simulink model "part19"  (R2017b)
settings: Solver=VariableStepAuto  StartTime=0.0  StopTime=40  RelTol=1e-3
settings Model: Creator=admin  LastModifiedBy=admin

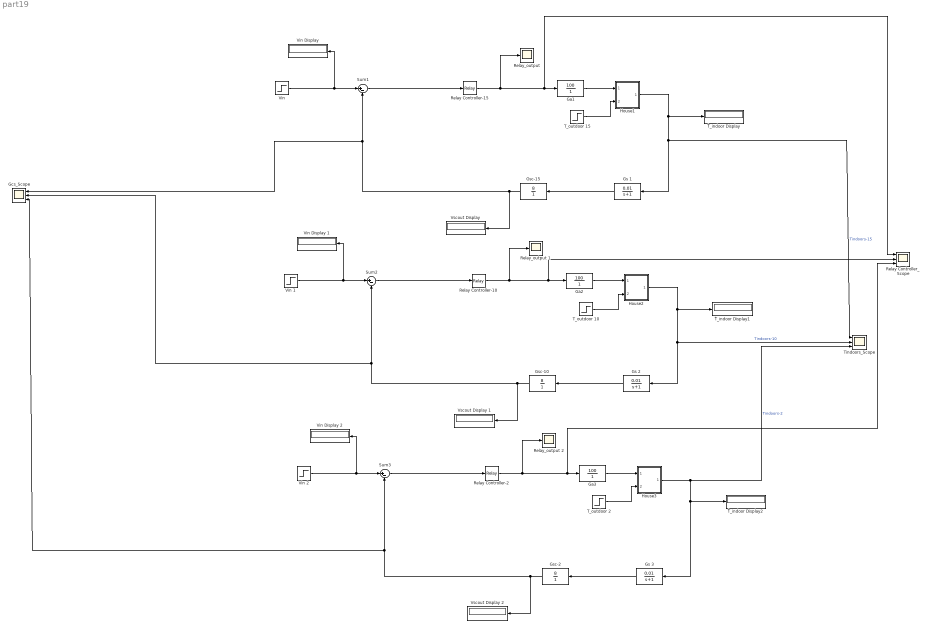
== system part19 ==
  Ga1 : TransferFcn  Numerator=[100]  Denominator=[1 ]
  Ga2 : TransferFcn  Numerator=[100]  Denominator=[1 ]
  Ga3 : TransferFcn  Numerator=[100]  Denominator=[1 ]
  "Gcs_Scope " : Scope  NumInputPorts=3
  Gs 1 : TransferFcn  Numerator=[0.01]  Denominator=[1 1]
  Gs 2 : TransferFcn  Numerator=[0.01]  Denominator=[1 1]
  Gs 3 : TransferFcn  Numerator=[0.01]  Denominator=[1 1]
  Gsc-10 : TransferFcn  Numerator=[8]  Denominator=[1 ]
  Gsc-15 : TransferFcn  Numerator=[8]  Denominator=[1 ]
  Gsc-2 : TransferFcn  Numerator=[8]  Denominator=[1 ]
  House1 : Subsystem
      mask Display: image(fullfile(matlabroot,'toolbox','simulink','simdemos','simgeneral','images','HouseHeatHousePix.svg'))
  House2 : Subsystem
      mask Display: image(fullfile(matlabroot,'toolbox','simulink','simdemos','simgeneral','images','HouseHeatHousePix.svg'))
  House3 : Subsystem
      mask Display: image(fullfile(matlabroot,'toolbox','simulink','simdemos','simgeneral','images','HouseHeatHousePix.svg'))
  Relay Controller-10 : Relay  OnSwitchValue=0.001  OffSwitchValue=-0.001  OnOutputValue=10
  Relay Controller-15 : Relay  OnSwitchValue=0.001  OffSwitchValue=-0.001  OnOutputValue=10
  Relay Controller-2 : Relay  OnSwitchValue=0.001  OffSwitchValue=-0.001  OnOutputValue=10
  "Relay Controller_Scope " : Scope  NumInputPorts=3
  "Relay_output " : Scope
  Relay_output 1 : Scope
  Relay_output 2 : Scope
  Sum1 : Sum  Inputs=|+-
  Sum2 : Sum  Inputs=|+-
  Sum3 : Sum  Inputs=|+-
  T_outdoor 10 : Step  Time=0  After=10  SampleTime=0
  "T_outdoor 15 " : Step  Time=0  After=15  SampleTime=0
  T_outdoor 2 : Step  Time=0  After=2  SampleTime=0
  "Tindoors_Scope " : Scope  NumInputPorts=3
  "Vin " : Step  Time=0  After=2.061  SampleTime=0
  Vin 1 : Step  Time=0  After=2.061  SampleTime=0
  Vin 2 : Step  Time=0  After=2.061  SampleTime=0
  "Vin Display " : Display
  Vin Display 1 : Display
  Vin Display 2 : Display
  "Vscout Display " : Display
  Vscout Display 1 : Display
  Vscout Display 2 : Display
  ْT_indoor Display : Display
  ْT_indoor Display1 : Display
  ْT_indoor Display2 : Display
  wires:
  "Vin "/1 -> "Vin Display "/1, Sum1/1
  Ga1/1 -> House1/1(Heater QDot In)
  Gs 1/1 -> Gsc-15/1
  Relay Controller-15/1 -> "Relay Controller_Scope "/1, Ga1/1, "Relay_output "/1
  Sum1/1 -> Relay Controller-15/1
  Gsc-15/1 -> "Gcs_Scope "/1, Sum1/2, "Vscout Display "/1
  "T_outdoor 15 "/1 -> House1/2(Outdoor Temp Tout)
  House1/1(Room Temp Troom) -> ْT_indoor Display/1, Gs 1/1, "Tindoors_Scope "/1  "Tindoors-15"
  Vin 1/1 -> Vin Display 1/1, Sum2/1
  Ga2/1 -> House2/1(Heater QDot In)
  Gs 2/1 -> Gsc-10/1
  Relay Controller-10/1 -> "Relay Controller_Scope "/2, Ga2/1, Relay_output 1/1
  Sum2/1 -> Relay Controller-10/1
  Gsc-10/1 -> "Gcs_Scope "/2, Sum2/2, Vscout Display 1/1
  T_outdoor 10/1 -> House2/2(Outdoor Temp Tout)
  House2/1(Room Temp Troom) -> ْT_indoor Display1/1, "Tindoors_Scope "/2, Gs 2/1  "Tindoors-10"
  Vin 2/1 -> Vin Display 2/1, Sum3/1
  Ga3/1 -> House3/1(Heater QDot In)
  Gs 3/1 -> Gsc-2/1
  Relay Controller-2/1 -> "Relay Controller_Scope "/3, Ga3/1, Relay_output 2/1
  Sum3/1 -> Relay Controller-2/1
  Gsc-2/1 -> "Gcs_Scope "/3, Sum3/2, Vscout Display 2/1
  T_outdoor 2/1 -> House3/2(Outdoor Temp Tout)
  House3/1(Room Temp Troom) -> "Tindoors_Scope "/3, ْT_indoor Display2/1, Gs 3/1  "Tindoors-2"

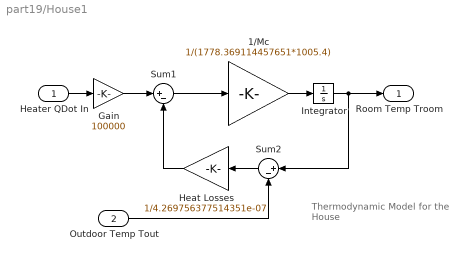
== system part19/House1 ==
  note: Thermodynamic Model
      | for the House
  Heater QDot In : Inport
  Outdoor Temp Tout : Inport  Port=2
  1/Mc : Gain  Gain=1/(1778.369114457651*1005.4)  SaturateOnIntegerOverflow=on  OutDataTypeStr=Inherit: Same as input  ParamDataTypeStr=Inherit: Same as input
  Gain : Gain  Gain=100000
  Heat Losses : Gain  Gain=1/4.269756377514351e-07  SaturateOnIntegerOverflow=on  OutDataTypeStr=Inherit: Same as input  ParamDataTypeStr=Inherit: Same as input
  Integrator : Integrator  InitialCondition=20
  Sum1 : Sum  Inputs=|+-  SaturateOnIntegerOverflow=on  InputSameDT=on  OutDataTypeStr=Inherit: Same as first input
  Sum2 : Sum  Inputs=|+-  SaturateOnIntegerOverflow=on  InputSameDT=on  OutDataTypeStr=Inherit: Same as first input
  Room Temp Troom : Outport  InitialOutput=0
  wires:
  Outdoor Temp Tout/1 -> Sum2/2
  Heater QDot In/1 -> Gain/1
  Sum1/1 -> 1/Mc/1
  Sum2/1 -> Heat Losses/1
  Heat Losses/1 -> Sum1/2
  1/Mc/1 -> Integrator/1
  Integrator/1 -> Sum2/1, Room Temp Troom/1
  Gain/1 -> Sum1/1

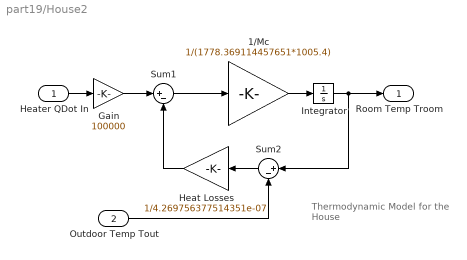
== system part19/House2 ==
  note: Thermodynamic Model
      | for the House
  Heater QDot In : Inport
  Outdoor Temp Tout : Inport  Port=2
  1/Mc : Gain  Gain=1/(1778.369114457651*1005.4)  SaturateOnIntegerOverflow=on  OutDataTypeStr=Inherit: Same as input  ParamDataTypeStr=Inherit: Same as input
  Gain : Gain  Gain=100000
  Heat Losses : Gain  Gain=1/4.269756377514351e-07  SaturateOnIntegerOverflow=on  OutDataTypeStr=Inherit: Same as input  ParamDataTypeStr=Inherit: Same as input
  Integrator : Integrator  InitialCondition=20
  Sum1 : Sum  Inputs=|+-  SaturateOnIntegerOverflow=on  InputSameDT=on  OutDataTypeStr=Inherit: Same as first input
  Sum2 : Sum  Inputs=|+-  SaturateOnIntegerOverflow=on  InputSameDT=on  OutDataTypeStr=Inherit: Same as first input
  Room Temp Troom : Outport  InitialOutput=0
  wires:
  Outdoor Temp Tout/1 -> Sum2/2
  Heater QDot In/1 -> Gain/1
  Sum1/1 -> 1/Mc/1
  Sum2/1 -> Heat Losses/1
  Heat Losses/1 -> Sum1/2
  1/Mc/1 -> Integrator/1
  Integrator/1 -> Sum2/1, Room Temp Troom/1
  Gain/1 -> Sum1/1

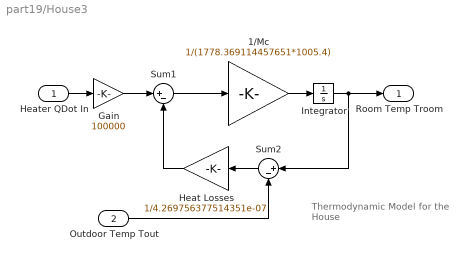
== system part19/House3 ==
  note: Thermodynamic Model
      | for the House
  Heater QDot In : Inport
  Outdoor Temp Tout : Inport  Port=2
  1/Mc : Gain  Gain=1/(1778.369114457651*1005.4)  SaturateOnIntegerOverflow=on  OutDataTypeStr=Inherit: Same as input  ParamDataTypeStr=Inherit: Same as input
  Gain : Gain  Gain=100000
  Heat Losses : Gain  Gain=1/4.269756377514351e-07  SaturateOnIntegerOverflow=on  OutDataTypeStr=Inherit: Same as input  ParamDataTypeStr=Inherit: Same as input
  Integrator : Integrator  InitialCondition=20
  Sum1 : Sum  Inputs=|+-  SaturateOnIntegerOverflow=on  InputSameDT=on  OutDataTypeStr=Inherit: Same as first input
  Sum2 : Sum  Inputs=|+-  SaturateOnIntegerOverflow=on  InputSameDT=on  OutDataTypeStr=Inherit: Same as first input
  Room Temp Troom : Outport  InitialOutput=0
  wires:
  Outdoor Temp Tout/1 -> Sum2/2
  Heater QDot In/1 -> Gain/1
  Sum1/1 -> 1/Mc/1
  Sum2/1 -> Heat Losses/1
  Heat Losses/1 -> Sum1/2
  1/Mc/1 -> Integrator/1
  Integrator/1 -> Sum2/1, Room Temp Troom/1
  Gain/1 -> Sum1/1
